simulink model "indy7_dualArm"  (R2024b)
settings: Solver=FixedStepAuto  StartTime=0.0  StopTime=10  FixedStep=0.001  RelTol=1e-3
model workspace (MAT data in the model file):
  joint_friction = [80 80 20 10 10 5]
  lambda_l_list = [0  -0.111945470246  -0.45  -0.23208429101  -0.00722667581655  -0.0911029490978  6.11257062428e-36; -1.17357539658  0.0246912114191  0  0.181466898367  -0.0447110760186  0.02862210596  -2.25514051877e-16; 0.993815552956  0.243747835972  -0.0305  0.141365128074  0.14506822671  0.174516399919  0.06; -2.091  1.20917417944  0  -1.20917417944  1.20917417944  -1.20917417944  0; 0  1.20917417944  0  -1.20905770917  1.20917417944  -1.20905770917  0; 0  -1.20905770917  0  1.20917417944  -1.20905770917  1.20917417944  0]
  lambda_r_list = [0  -0.111945470246  -0.45  -0.23208429101  -0.00722667581655  -0.0911029490978  -2.58853268681e-20; 1.17618914658  0.0246912114191  1.73472347598e-18  0.181466898367  -0.0447110760186  0.02862210596  2.25514051877e-16; 0.992300581915  0.243747835972  -0.0305  0.141365128074  0.14506822671  0.174516399919  0.06; 2.091  1.20917417944  1.04335921902e-16  -1.20917417944  1.20917417944  -1.20917417944  -1.83339582048e-16; 0  1.20917417944  -5.59082217244e-17  -1.20905770917  1.20917417944  -1.20905770917  -4.06575814682e-20; 0  -1.20905770917  1.31751732896e-17  1.20917417944  -1.20905770917  1.20917417944  0]
  lambda_rl_list = [2.58853268681e-20  0.0911029490978  0.00722667581655  0.23208429101  0.45  0.111945470246  0.701934663685  -0.111945470246  -0.45  -0.23208429101  -0.00722667581655  -0.0911029490978  2.43945488809e-21; -2.25514051877e-16  -0.02862210596  0.0447110760186  -0.181466898367  -1.73472347598e-18  -0.0246912114191  -0.00107834177066  0.0246912114191  -1.03338019565e-22  0.181466898367  -0.0447110760186  0.02862210596  -2.11636264069e-16; -0.06  -0.174516399919  -0.14506822671  -0.141365128074  0.0305  -0.243747835972  0.00061752626027  0.243747835972  -0.0305  0.141365128074  0.14506822671  0.174516399919  0.06; -1.83339582048e-16  1.20917417944  -1.20917417944  1.20917417944  1.04335921902e-16  -1.20917417944  -8.63118783402e-10  1.20917417944  0  -1.20917417944  1.20917417944  -1.20917417944  -2.89997910743e-16; -4.06575814682e-20  1.20905770917  -1.20917417944  1.20905770917  -5.59082217244e-17  -1.20917417944  2.72601580299  1.20917417944  -3.44383110592e-41  -1.20905770917  1.20917417944  -1.20905770917  -8.13151629364e-20; 0  -1.20917417944  1.20905770917  -1.20917417944  1.31751732896e-17  1.20905770917  -1.56154991477  -1.20905770917  0  1.20917417944  -1.20905770917  1.20917417944  0]
  q_init_l = Simulink.Parameter
  q_init_l.Value = [0.165747; 0.819274; 1.26369; 0.604148; 1.0515; -0.139217]
  q_init_l.Complexity = 'real'
  q_init_l.Dimensions = [6 1]
  q_init_l.DataType = 'double'
  q_init_l1 = Simulink.Parameter
  q_init_l1.Value = 0.165747
  q_init_l1.Complexity = 'real'
  q_init_l1.Dimensions = [1 1]
  q_init_l1.DataType = 'double'
  q_init_l2 = Simulink.Parameter
  q_init_l2.Value = 0.819274
  q_init_l2.Complexity = 'real'
  q_init_l2.Dimensions = [1 1]
  q_init_l2.DataType = 'double'
  q_init_l3 = Simulink.Parameter
  q_init_l3.Value = 1.26369
  q_init_l3.Complexity = 'real'
  q_init_l3.Dimensions = [1 1]
  q_init_l3.DataType = 'double'
  q_init_l4 = Simulink.Parameter
  q_init_l4.Value = 0.604148
  q_init_l4.Complexity = 'real'
  q_init_l4.Dimensions = [1 1]
  q_init_l4.DataType = 'double'
  q_init_l5 = Simulink.Parameter
  q_init_l5.Value = 1.0515
  q_init_l5.Complexity = 'real'
  q_init_l5.Dimensions = [1 1]
  q_init_l5.DataType = 'double'
  q_init_l6 = Simulink.Parameter
  q_init_l6.Value = -0.139217
  q_init_l6.Complexity = 'real'
  q_init_l6.Dimensions = [1 1]
  q_init_l6.DataType = 'double'
  q_init_r = Simulink.Parameter
  q_init_r.Value = [-0.165747; -0.819274; -1.26369; -0.604148; -1.0515; 0.139217]
  q_init_r.Complexity = 'real'
  q_init_r.Dimensions = [6 1]
  q_init_r.DataType = 'double'
  q_init_r1 = Simulink.Parameter
  q_init_r1.Value = -0.165747
  q_init_r1.Complexity = 'real'
  q_init_r1.Dimensions = [1 1]
  q_init_r1.DataType = 'double'
  q_init_r2 = Simulink.Parameter
  q_init_r2.Value = -0.819274
  q_init_r2.Complexity = 'real'
  q_init_r2.Dimensions = [1 1]
  q_init_r2.DataType = 'double'
  q_init_r3 = Simulink.Parameter
  q_init_r3.Value = -1.26369
  q_init_r3.Complexity = 'real'
  q_init_r3.Dimensions = [1 1]
  q_init_r3.DataType = 'double'
  q_init_r4 = Simulink.Parameter
  q_init_r4.Value = -0.604148
  q_init_r4.Complexity = 'real'
  q_init_r4.Dimensions = [1 1]
  q_init_r4.DataType = 'double'
  q_init_r5 = Simulink.Parameter
  q_init_r5.Value = -1.0515
  q_init_r5.Complexity = 'real'
  q_init_r5.Dimensions = [1 1]
  q_init_r5.DataType = 'double'
  q_init_r6 = Simulink.Parameter
  q_init_r6.Value = 0.139217
  q_init_r6.Complexity = 'real'
  q_init_r6.Dimensions = [1 1]
  q_init_r6.DataType = 'double'
  robot : robotics.RigidBodyTree (value not decoded)
values from neighbouring files (symbols this model uses):
  lambda_lr_list = [lambda_lr_list,-lambda_rl_list(:,i)]    [getDualArmLambdaList.m]    (also in untitled3.m)
  m = models{k}    [code_generation.m]
  N = length(q)    [FKLocalPOE.m]
undefined symbols (not defined in the file or in its folder): Blist_tcp, DiscIntNeverNeededParam, dt, exp6, M_tcp, q_init, q_max, q_min, qdot_max, qdot_min, SW_a, SW_b0, X, Y, Z
libraries: sm_lib x148, nesl_utility x45, robotmaniplib x9, robotcorelib x5, simulink x4, matrix_library x2
(part 1 of 5)
settings Model: Creator=sung  LastModifiedBy=sung
settings ExplorerConfigSet: InternalSimMechanicsExplorerSettings="<ExplorerConfiguration><canonicalview>default</canonicalview><AnimationSetting><BasePlaybackSpeed>1.0</BasePlaybackSpeed><PlaybackSpeedFactor>1.0</PlaybackSpeedFactor></AnimationSetting><TilePanel><TileInfo><Tiles Columns=\"1\" Count=\"1\" Rows=\"1\"><Column Weight=\"1\"/><Row Weight=\"1\"/><Tile Height=\"1\" Width=\"1\" X=\"0\" Y=\"0\"/></Tiles></TileInfo><SceneInfo><SceneViewer><BGColor><R>1</R><G>1</G><B>1</B></BGColor><Camera><DoPerspective>off</DoPerspective><Position><X>1.65343822930104345</X><Y>-0.838028370601997863</Y><Z>1.3090619282042868</Z></Position><Center><X>0.667257287193148252</X><Y>-0.49026343910033765</Y><Z>0.88933438419422528</Z></Center><Up><X>-0.446910653050087703</X><Y>-0.221156484844483803</Y><Z>0.866810635260998552</Z></Up><ViewLimDist>1</ViewLimDist><YLim>0.778338166596068581</YLim><XLim>1.03312002337695397</XLim></Camera></SceneViewer></SceneInfo></TilePanel><MechEditorPanel><Cameras/><GfxPanelCameraMap/><VideoCreator><PlaybackSpeedRatio>1.0</PlaybackSpeedRatio><FrameRate>30</FrameRate><VideoFormat>Motion JPEG AVI</VideoFormat><FrameSize>auto</FrameSize></VideoCreator></MechEditorPanel></ExplorerConfiguration>"

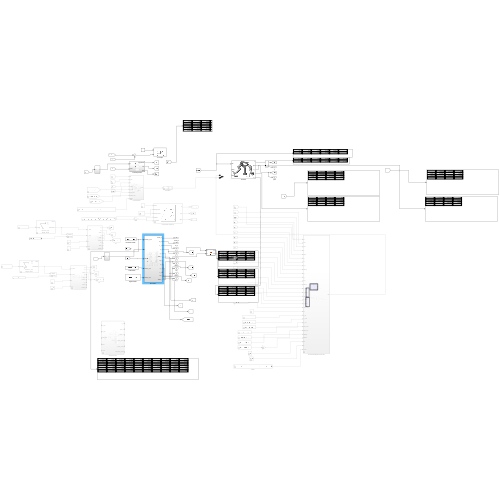
[thumbnail: Simulink's stored preview of the top-level diagram]
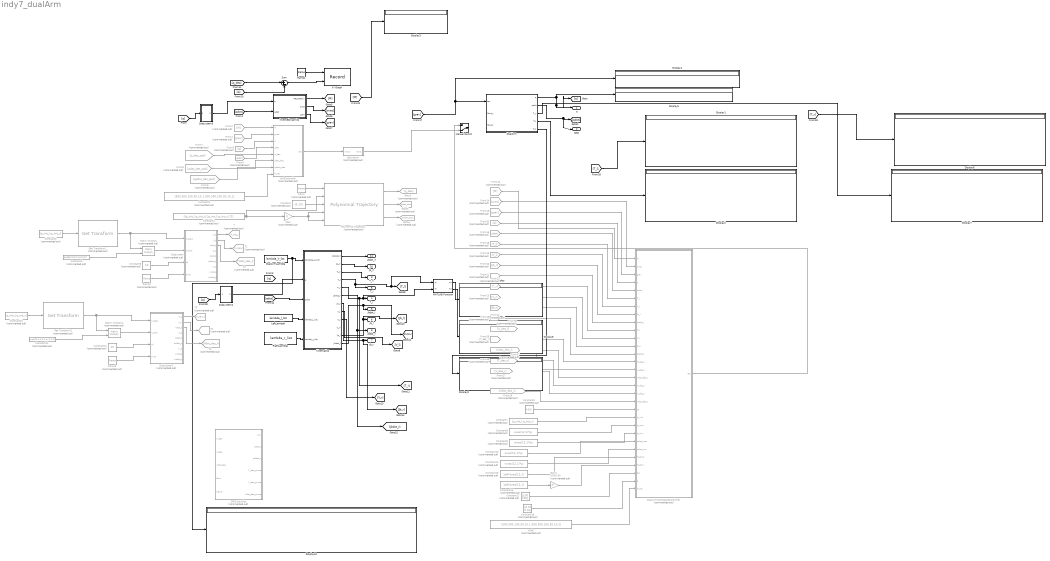
== system indy7_dualArm ==
  Constant : Constant  Commented=on  Value=[0,10]
  Constant1 : Constant  Commented=on  Value=[[q_init_l;q_init_r],[q_init_l;q_init_r].*2]
  Constant10 : Constant  Commented=on  Value=[q_init_l;q_init_r]
  Constant11 : Constant  Commented=on  Value=exp6([0.1,0,0.1,pi/2,0,0]')
  Constant12 : Constant  Commented=on  Value=10
  Constant13 : Constant  Commented=on  Value=ones(12,1)*pi
  Constant14 : Constant  Commented=on  Value=-ones(12,1)*pi
  Constant15 : Constant  Commented=on  Value=1e6*ones(12,1)
  Constant16 : Constant  Commented=on  Value=1e6*ones(12,1)
  Constant17 : Constant  Commented=on  Value=[100 100]
  Constant18 : Constant  Commented=on  Value=[0.01 0.01]
  Constant2 : Constant  Commented=on  Value=[500,500,100,50,10,1,500,500,100,50,10,1]
  Constant3 : Constant  Commented=on  Value=[q_init_l;q_init_r]
  Constant4 : Constant  Commented=on  Value=exp6([0,0,0.1,0,0,0]')
  Constant5 : Constant  Commented=on  Value=10
  Constant6 : Constant  Commented=on  Value=0.001
  Constant7 : Constant  Commented=on  Value=[q_init_l;q_init_r]
  Constant8 : Constant  Commented=on  Value=ones(12,1)*pi
  Constant9 : Constant  Commented=on  Value=-ones(12,1)*pi
  Display{,1..10} (11 alike) : Display
  DualArm : Subsystem
      mask Display: image('dualarm.png');
  DualArmLambda : Constant  Value=lambda_lr_list
  DualArmTaskSpaceController : Subsystem  Commented=on
  From13 : From  Commented=on  GotoTag=M
  From14 : From  Commented=on  GotoTag=cvec
  From15 : From  Commented=on  GotoTag=grav
  From16 : From  Commented=on  GotoTag=qdot
  From18 : From  Commented=on  GotoTag=T_l
  From19 : From  Commented=on  GotoTag=V_l
  From2 : From  Commented=on  GotoTag=M
  From20 : From  Commented=on  GotoTag=Jb_l
  From21 : From  Commented=on  GotoTag=Jbdot_l
  From22 : From  Commented=on  GotoTag=T_r
  From23 : From  Commented=on  GotoTag=V_r
  From24 : From  Commented=on  GotoTag=Jb_r
  From25 : From  Commented=on  GotoTag=Jbdot_r
  From26 : From  Commented=on  GotoTag=T_des_l
  From27 : From  Commented=on  GotoTag=V_des_r
  From29 : From  Commented=on  GotoTag=Vdot_des_r
  From32 : From  Commented=on  GotoTag=q
  From36 : From  Commented=on  GotoTag=V_des_l
  From37 : From  Commented=on  GotoTag=Vdot_des_l
  From38 : From  Commented=on  GotoTag=T_des_r
  From4 : From  Commented=on  GotoTag=grav
  From5 : From  Commented=on  GotoTag=q
  From6 : From  Commented=on  GotoTag=qdot
  From7 : From  Commented=on  GotoTag=q_des_spd
  From8 : From  Commented=on  GotoTag=qdot_des_spd
  From9 : From  Commented=on  GotoTag=qddot_des_spd
  Gain : Gain  Commented=on  Gain=0
  Gain1 : Gain  Commented=on  Gain=0.001*30
  Get Transform1 : robotmaniplib/Get Transform  Commented=on  RigidBodyTree=robot  SourceBody=l_tcp  TargetBody=world  SimulateUsing=Code generation
  Get Transform2 : robotmaniplib/Get Transform  Commented=on  RigidBodyTree=robot  SourceBody=r_tcp  TargetBody=world  SimulateUsing=Code generation
  Goto2 : Goto  Commented=on  GotoTag=q_des
  Goto3 : Goto  Commented=on  GotoTag=qdot_des
  Goto4 : Goto  Commented=on  GotoTag=qddot_des
  HInfController : Subsystem  Commented=on
  HinfK : Constant  Commented=on  Value=[500,500,100,50,10,1,500,500,100,50,10,1]
  InverseDynamics : Subsystem
  Kinematics : Subsystem
  LeftLambda : Constant  Value=lambda_l_list
  MATLAB Function : MATLAB Function  TreatAsAtomicUnit=on
  Manual Switch : ManualSwitch  CurrentSetting=0
  Matrix Multiply : Product  Commented=on  Multiplication=Matrix(*)
  Matrix Multiply1 : Product  Commented=on  Multiplication=Matrix(*)
  Polynomial Trajectory : robotcorelib/Polynomial Trajectory  Commented=on  WaypointSource=External  Waypoints=[ 0, 2, 1, 5, 0; -1, 3, 1, 4, 4 ]  TimePoints=[ 0, 1, 2, 3, 4 ]  TimeInterval=[ 1, 4 ]  Method=Quintic Polynomial  ParameterSource=External  VelocityBoundaryCondition=zeros( 2, 5 )  AccelerationBoundaryCondition=zeros( 2, 5 )  SimulateUsing=Interpreted execution
  Ramp : simulink/Sources/Ramp  Commented=on  slope=1  start=0  InitialOutput=0
  Ramp1 : simulink/Sources/Ramp  slope=1  start=0  InitialOutput=0
  Ramp2 : simulink/Sources/Ramp  Commented=on  slope=1  start=0  InitialOutput=0
  Ramp3 : simulink/Sources/Ramp  Commented=on  slope=1  start=0  InitialOutput=0
  RightLambda : Constant  Value=lambda_r_list
  SPDController : Subsystem  Commented=on
  Saturation : Subsystem  Commented=on
  Subsystem : Subsystem  Commented=on
  Subsystem1 : Subsystem  Commented=on
  Subsystem2 : Subsystem
  Subsystem3 : Subsystem
  Sum : Sum  Inputs=|+-
  T : Goto  Commented=on  GotoTag=T_des_l
  T1 : Goto  Commented=on  GotoTag=V_des_l
  T2 : Goto  Commented=on  GotoTag=Vdot_des_l
  T3 : Goto  Commented=on  GotoTag=T_des_r
  T4 : Goto  Commented=on  GotoTag=V_des_r
  T5 : Goto  Commented=on  GotoTag=Vdot_des_r
  XY Graph : Record  FileSettingsInternal="{\"entries\":[{\"content\":{\"excelSettings\":{\"content\":{},\"type\":\"Streamout.ExcelSettings\"}},\"type\":\"Streamout.FileSettingStorage\",\"uuid\":\"\"}],\"packageUris\":[\"http:\\/\\/schema.mathworks.com\\/mf0\\/streamout_blocks\\/R2020a\"],\"version\":\"1.0\"}"  Layout=[1 1]  SignalsInternal="{\"entries\":[{\"content\":{\"signals\":[{\"content\":{\"blockPath\":[],\"dimensions\":[1],\"domain\":\"\",\"lineColor\":\"#a2142f\",\"plots\":[ 1 ],\"port\":1,\"sid\":[\"\"],\"signalID\":1,\"signalName\":\"Ramp1\"},\"type\":\"RecordBlkView.Signal\",\"uuid\":\"\"},{\"content\":{\"blockPath\":[],\"dimensions\":[12],\"domain\":\"\",\"hasChildren\":true,\"lineColor\":\"#77ac30\",\"lineWidth\":2,\"port\":2,\"sid\":[\"\"],\"signalID\":2,\"signalName\":\"Sum\"},\"type\":\"RecordBlkView.Signal\",\"uuid\":\"\"},{\"content\":{\"blockPath\":[],\"channel\":[1],\"dimensions\":[12],\"domain\":\"\",\"lineColor\":\"#77ac30\",\"lineWidth\":2,\"parentID\":2,\"port\":2,\"sid\":[\"\"],\"signalID\":3,\"signalName\":\"Sum\"},\"type\":\"RecordBlkView.Signal\",\"uuid\":\"\"}]},\"type\":\"RecordBlkView.InputSignals\",\"uuid\":\"\"}],\"packageUris\":[\"http:\\/\\/schema.mathworks.com\\/mf0\\/streamout_blocks\\/R2020a\"],\"version\":\"1.0\"}"  VisualizationBindings="{\"xyplotplugin\":{\"info\":[{\"series\":[{\"bindingParametersList\":[{\"parameter\":\"X-Axis\",\"signalID\":1,\"signalName\":\"Ramp1\"}],\"seriesID\":0},{\"bindingParametersList\":[{\"parameter\":\"X-Axis\",\"signalID\":1,\"signalName\":\"Ramp1\"}],\"seriesID\":1},{\"bindingParametersList\":[{\"parameter\":\"X-Axis\",\"signalID\":1,\"signalName\":\"Ramp1\"}],\"seriesID\":2},{\"bindingParametersList\":[{\"parameter\":\"X-Axis\",\"signalID\":1,\"signalName\":\"Ramp1\"}],\"seriesID\":3},{\"bindingParametersList\":[{\"parameter\":\"X-Axis\",\"signalID\":1,\"signalName\":\"Ramp1\"}],\"seriesID\":4},{\"bindingParametersList\":[{\"parameter\":\"X-Axis\",\"signalID\":1,\"signalName\":\"Ramp1\"}],\"seriesID\":5},{\"bindingParametersList\":[{\"parameter\":\"X-Axis\",\"signalID\":1,\"signalName\":\"Ramp1\"}],\"seriesID\":6},{\"bindingParametersList\":[{\"parameter\":\"X-Axis\",\"signalID\":1,\"signalName\":\"Ramp1\"}],\"seriesID\":7},{\"bindingParametersList\":[{\"parameter\":\"X-Axis\",\"signalID\":1,\"signalName\":\"Ramp1\"}],\"seriesID\":8},{\"bindingParametersList\":[{\"parameter\":\"X-Axis\",\"signalID\":1,\"signalName\":\"Ramp1\"}],\"seriesID\":9},{\"bindingParametersList\":[{\"parameter\":\"X-Axis\",\"signalID\":1,\"signalName\":\"Ramp1\"}],\"seriesID\":10}],\"subplotID\":1}]}}"  CompatibilityTag=XY
  q : Outport
  qdot : Outport  Port=2
  T_rl : Outport  Port=3
  T_r : Outport  Port=4
  T_l : Outport  Port=5
  Jb_l : Outport  Port=6
  Jb_r : Outport  Port=7
  Jbdot_l : Outport  Port=8
  Jbdot_r : Outport  Port=9
  Jb_rl : Outport  Port=10
  Jbdot_rl : Outport  Port=11
  wires:
  InverseDynamics/3(grav) -> [grav]
  [q_des] -> Sum/1
  From2/1 -> HInfController/1(M)
  DualArm/2(qdot) -> qdot/1, [qdot]
  [q] -> Sum/2
  From5/1 -> HInfController/3(q)
  [qdot] -> InverseDynamics/2(qdot)
  From4/1 -> HInfController/2(gvec)
  From6/1 -> HInfController/4(qdot)
  From7/1 -> HInfController/5(q_des)
  From8/1 -> HInfController/6(qdot_des)
  From9/1 -> HInfController/7(qddot_des)
  InverseDynamics/1(MassMatrix) -> [M]
  Constant1/1 -> Polynomial Trajectory/2, Gain/1
  Constant2/1 -> HInfController/8(HinfK)
  Ramp1/1 -> XY Graph/1
  Sum/1 -> XY Graph/2
  InverseDynamics/2(cvec) -> [cvec]
  HInfController/1(tau) -> Saturation/1(Input)
  Ramp/1 -> Polynomial Trajectory/1
  Polynomial Trajectory/2 -> Goto3/1
  Constant/1 -> Polynomial Trajectory/3
  Gain/1 -> Polynomial Trajectory/5, Polynomial Trajectory/4
  Polynomial Trajectory/1 -> Goto2/1
  Polynomial Trajectory/3 -> Goto4/1
  DualArm/1(q) -> [q], q/1, Display5/1
  DualArmLambda/1 -> Display10/1, Kinematics/1(lambda_lr_list)
  [qdot] -> Kinematics/3(qdot)
  Kinematics/1(Jbdot_lrl) -> Jbdot_rl/1
  Kinematics/2(Jb_lr) -> Jb_rl/1
  Kinematics/3(T_lr) -> T_rl/1
  Kinematics/4(T_l) -> T_l/1, MATLAB Function/1(Tl), [T_l]
  Kinematics/5(T_r) -> [T_r], MATLAB Function/2(Tr), T_r/1
  Kinematics/12(Jbdot_l) -> Jbdot_l/1, [Jbdot_l]
  Kinematics/11(Jb_l) -> [Jb_l], Jb_l/1
  Kinematics/6(Jbdot_r) -> [Jbdot_r], Jbdot_r/1
  Kinematics/7(Jb_r) -> [Jb_r], Jb_r/1
  LeftLambda/1 -> Kinematics/4(lamba_l_list)
  RightLambda/1 -> Kinematics/5(lamba_r_list)
  Constant3/1 -> Get Transform1/1
  Get Transform1/1 -> Matrix Multiply/1, Subsystem/1(T_start)
  Constant4/1 -> Matrix Multiply/2
  Matrix Multiply/1 -> Subsystem/2(T_end)
  Constant5/1 -> Subsystem/3(Tf)
  Ramp2/1 -> Subsystem/4(time)
  Subsystem/1(T_t) -> T/1
  Subsystem/2(V_t) -> T1/1
  Subsystem/3(Vdot_t) -> T2/1
  Kinematics/8(V_l) -> [V_l]
  Subsystem1/2(V_t) -> T4/1
  Ramp3/1 -> Subsystem1/4(time)
  Subsystem1/3(Vdot_t) -> T5/1
  Constant10/1 -> Get Transform2/1
  Matrix Multiply1/1 -> Subsystem1/2(T_end)
  Constant11/1 -> Matrix Multiply1/2
  Get Transform2/1 -> Matrix Multiply1/1, Subsystem1/1(T_start)
  Constant12/1 -> Subsystem1/3(Tf)
  Subsystem1/1(T_t) -> T3/1
  Kinematics/9(V_r) -> [V_r]
  Saturation/1(Out1) -> Manual Switch/2
  From13/1 -> DualArmTaskSpaceController/1(M)
  From14/1 -> DualArmTaskSpaceController/2(cvec)
  From15/1 -> DualArmTaskSpaceController/3(grav)
  From32/1 -> DualArmTaskSpaceController/4(q)
  From16/1 -> DualArmTaskSpaceController/5(qdot)
  Constant6/1 -> DualArmTaskSpaceController/20(dt)
  From18/1 -> DualArmTaskSpaceController/6(T_l)
  From19/1 -> DualArmTaskSpaceController/7(V_l)
  From20/1 -> DualArmTaskSpaceController/8(Jb_l)
  From21/1 -> DualArmTaskSpaceController/9(Jbdot_l)
  From22/1 -> DualArmTaskSpaceController/10(T_r)
  From23/1 -> DualArmTaskSpaceController/11(V_r)
  From24/1 -> DualArmTaskSpaceController/12(Jb_r)
  From25/1 -> DualArmTaskSpaceController/13(Jbdot_r)
  From26/1 -> DualArmTaskSpaceController/14(T_des_l)
  From36/1 -> DualArmTaskSpaceController/15(V_des_l)
  From37/1 -> DualArmTaskSpaceController/16(Vdot_des_l)
  From38/1 -> DualArmTaskSpaceController/17(T_des_r)
  From27/1 -> DualArmTaskSpaceController/18(V_des_r)
  From29/1 -> DualArmTaskSpaceController/19(Vdot_des_r)
  Constant7/1 -> DualArmTaskSpaceController/21(q_init)
  Constant8/1 -> DualArmTaskSpaceController/22(q_max)
  Constant9/1 -> DualArmTaskSpaceController/23(q_min)
  Constant13/1 -> DualArmTaskSpaceController/24(qdot_max)
  Constant14/1 -> DualArmTaskSpaceController/25(qdot_min)
  Constant15/1 -> DualArmTaskSpaceController/26(TaskKp)
  Constant16/1 -> Gain1/1
  Gain1/1 -> DualArmTaskSpaceController/27(TaskKv)
  Constant17/1 -> DualArmTaskSpaceController/28(b0)
  Constant18/1 -> DualArmTaskSpaceController/29(a)
  HinfK/1 -> DualArmTaskSpaceController/30(HinfK)
  DualArmTaskSpaceController/1(tau) -> Manual Switch/1
  MATLAB Function/1(Tlr) -> Display/1
  [grav] -> Display4/1, DualArm/1(tau)
  [T_l] -> Display1/1
  DualArm/4(T_l) -> Display2/1
  [q] -> Subsystem2/1(In1)
  Subsystem2/1(Out1) -> Kinematics/2(q)
  [M] -> Display3/1
  [q] -> Subsystem3/1(In1)
  Subsystem3/1(Out1) -> InverseDynamics/1(q)
  [T_r] -> Display6/1
  DualArm/3(T_r) -> Display7/1
  MATLAB Function/2(Trl) -> Display8/1
  DualArm/5(T_rl) -> Display9/1

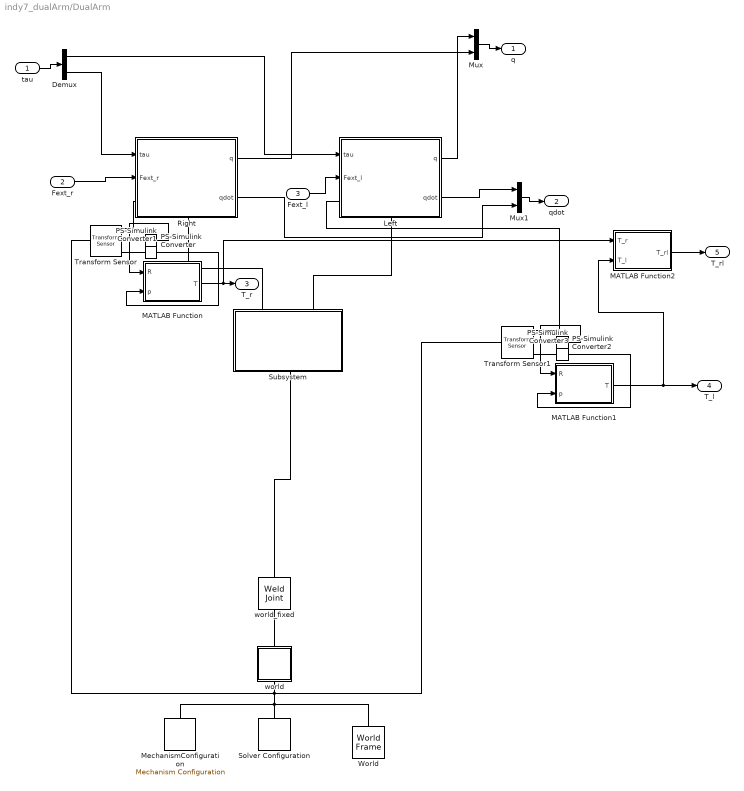
== system indy7_dualArm/DualArm ==
  tau : Inport
  Fext_r : Inport  Port=2
  Fext_l : Inport  Port=3
  Demux : Demux  Outputs=2
  Left : Subsystem
      settings: PortSchema="{\"entries\":[{\"content\":{\"sides\":[{\"content\":{\"connectorIds\":[\"In1\",\"In2\",\"LConn1\"]},\"type\":\"ConnectorPlacement.EquallySpacedRectSide\",\"uuid\":\"a802bf1d-865c-44a2-b0f5-a6da758969a6\"},{\"content\":{\"connectorIds\":[\"Out1\",\"Out2\"],\"side\":\"RIGHT\"},\"type\":\"ConnectorPlacement.EquallySpacedRectSide\",\"uuid\":\"5f6dd1c3-913e-4ce9-9167-95590779c30f\"},{\"content\":{\"side\":\"TOP\"},\"type\":\"ConnectorPlacement.EquallySpacedRectSide\",\"uuid\":\"64c6b8e9-73c0-45a3-a4f2-c2cb7725a77f\"},{\"content\":{\"connectorIds\":[\"RConn1\"],\"side\":\"BOTTOM\"},\"type\":\"ConnectorPlacement.EquallySpacedRectSide\",\"uuid\":\"95edfb6b-d02c-40cc-a449-2c9849400bda\"}]},\"type\":\"ConnectorPlacement.EquallySpacedConnector\",\"uuid\":\"45caad31-32a3-4e19-8c7b-99b9e1313351\"}],\"packageUris\":[\"http://schema.mathworks.com/mf0/Connector/R2020b\"],\"version\":\"1.0\"}"
  MATLAB Function : MATLAB Function  TreatAsAtomicUnit=on
  MATLAB Function1 : MATLAB Function  TreatAsAtomicUnit=on
  MATLAB Function2 : MATLAB Function  TreatAsAtomicUnit=on
  MechanismConfiguration : sm_lib/Utilities/Mechanism Configuration  UniformGravity=Constant  GravityVector=[0 0 -9.80665]  GravityVectorUnits=m/s^2  LinearizationDelta=0.001  JointModeTransitionNonlinearIterations=2
  Mux : Mux  Inputs=2
  Mux1 : Mux  Inputs=2
  PS-Simulink Converter{,1..3} (4 alike) : nesl_utility/PS-Simulink Converter  PhysicalDomain=network_engine_domain  SubClassName=ps_output  LeftPortType=input  RightPortType=output  PseudoPeriodic=off  Frequencies=[]  VectorFormat=inherit  Unit=inherit  AffineConversion=off
  Right : Subsystem
      settings: PortSchema="{\"entries\":[{\"content\":{\"sides\":[{\"content\":{\"connectorIds\":[\"In1\",\"In2\",\"LConn1\"]},\"type\":\"ConnectorPlacement.EquallySpacedRectSide\",\"uuid\":\"fdf178f2-e7c3-4173-86ca-7321804fb5d5\"},{\"content\":{\"connectorIds\":[\"Out1\",\"Out2\"],\"side\":\"RIGHT\"},\"type\":\"ConnectorPlacement.EquallySpacedRectSide\",\"uuid\":\"59022458-aa9c-4c83-9b4f-7726f2382bb8\"},{\"content\":{\"side\":\"TOP\"},\"type\":\"ConnectorPlacement.EquallySpacedRectSide\",\"uuid\":\"4f63f239-705d-4500-8a4d-d984146f717c\"},{\"content\":{\"connectorIds\":[\"RConn1\"],\"side\":\"BOTTOM\"},\"type\":\"ConnectorPlacement.EquallySpacedRectSide\",\"uuid\":\"092b85dc-93e6-45d5-b73f-7a2a4320a625\"}]},\"type\":\"ConnectorPlacement.EquallySpacedConnector\",\"uuid\":\"427c422a-fe45-4c4a-9206-8f07c894b426\"}],\"packageUris\":[\"http://schema.mathworks.com/mf0/Connector/R2020b\"],\"version\":\"1.0\"}"
  Solver Configuration : nesl_utility/Solver Configuration  PhysicalDomain=network_engine_domain  SubClassName=solver  LeftPortType=input  RightPortType=generic  Tones=[]  Harmonics=[]  SimulateNoise=off  Profile=off  UseLocalSampling=off  EnableSwitchedLinearOptims=on  FrequencyDomain=off  UseCCode=off  RelTol=0.001  AbsTol=0.001  MinStep=1e-09  ToWorkspace=off  RevertToSquareIcSolve=off  NumHomotopyIterations=100  PhasorMode=off  PhasorModeNumHarmonics=1  ConsistencySolver=NEWTON_XTOL_AFTER_FTOL  IndexReductionMethod=DerivativeReplacement  DoDC=off  ResidualTolerance=1e-09  ConsistencyTolSource=GLOBAL  ConsistencyAbsTol=0.001  ConsistencyRelTol=0.001  ConsistencyTolFactor=0.001  UseLocalSolver=off  LocalSolverChoice=NE_BACKWARD_EULER_ADVANCER  ResolveIndetEquations=on  FunctionEvalNumThread=1  LocalSolverSampleTime=0.001  DoFixedCost=off  MaxNonlinIter=3  MaxModeIter=2  ComputeImpulses=off  ImpulseIterations=2  LinearAlgebra=auto  LinearAlgebraNumThread=0  EquationFormulation=NE_TIME_EF  DelaysMemoryBudget=1024  AutomaticFiltering=on  FilteringTimeConstant=0.001  PartitionStorageMethod=AS_NEEDED  PartitionMemoryBudget=1024  PartitionMethod=ROBUST  MultibodyUseLocalSolver=on  MultibodyLocalSolverChoice=ODE1  MultibodyLocalSolverSampleTime=0.001
  Subsystem : Subsystem
  Transform Sensor : sm_lib/Frames and Transforms/Transform Sensor  MeasurementFrame=World  RotationSequence=XYX  SenseAngle=off  SenseAxis=off  SenseQ=off  SenseR=on  SenseRotationSequence=off  SenseOmegaX=off  SenseOmegaY=off  SenseOmegaZ=off  SenseOmega=off  SenseQDot=off  SenseRDot=off  SenseRotationSequenceDot=off  SenseAlphaX=off  SenseAlphaY=off  SenseAlphaZ=off  SenseAlpha=off  SenseQDDot=off  SenseRDDot=off  SenseX=off  SenseY=off  SenseZ=off  SenseXYZ=on  SenseRad=off  SenseAzim=off  SenseDist=off  SenseInc=off  SenseXDot=off  SenseYDot=off  SenseZDot=off  SenseXYZDot=off  SenseRadDot=off  SenseAzimDot=off  SenseDistDot=off  SenseIncDot=off  SenseXDDot=off  SenseYDDot=off  SenseZDDot=off  SenseXYZDDot=off  SenseRadDDot=off  SenseAzimDDot=off  SenseDistDDot=off  SenseIncDDot=off
  Transform Sensor1 : sm_lib/Frames and Transforms/Transform Sensor  MeasurementFrame=World  RotationSequence=XYX  SenseAngle=off  SenseAxis=off  SenseQ=off  SenseR=on  SenseRotationSequence=off  SenseOmegaX=off  SenseOmegaY=off  SenseOmegaZ=off  SenseOmega=off  SenseQDot=off  SenseRDot=off  SenseRotationSequenceDot=off  SenseAlphaX=off  SenseAlphaY=off  SenseAlphaZ=off  SenseAlpha=off  SenseQDDot=off  SenseRDDot=off  SenseX=off  SenseY=off  SenseZ=off  SenseXYZ=on  SenseRad=off  SenseAzim=off  SenseDist=off  SenseInc=off  SenseXDot=off  SenseYDot=off  SenseZDot=off  SenseXYZDot=off  SenseRadDot=off  SenseAzimDot=off  SenseDistDot=off  SenseIncDot=off  SenseXDDot=off  SenseYDDot=off  SenseZDDot=off  SenseXYZDDot=off  SenseRadDDot=off  SenseAzimDDot=off  SenseDistDDot=off  SenseIncDDot=off
  World : sm_lib/Frames and Transforms/World Frame
  world : Subsystem
  world_fixed : sm_lib/Joints/Weld Joint  JointMode=Normal  CompositeWrenchDir=FollowerOnBase  CompositeWrenchFrame=BaseFrame  SenseConstraintForce=off  SenseConstraintTorque=off  SenseTotalForce=off  SenseTotalTorque=off
  q : Outport
  qdot : Outport  Port=2
  T_r : Outport  Port=3
  T_l : Outport  Port=4
  T_rl : Outport  Port=5
  wires:
  tau/1 -> Demux/1
  Left/1(q) -> Mux/1
  Mux/1 -> q/1
  Demux/2 -> Right/1(tau)
  Left/2(qdot) -> Mux1/1
  Mux1/1 -> qdot/1
  Right/1(q) -> Mux/2
  Right/2(qdot) -> Mux1/2
  Demux/1 -> Left/1(tau)
  PS-Simulink Converter/1 -> MATLAB Function/1(R)
  PS-Simulink Converter1/1 -> MATLAB Function/2(p)
  MATLAB Function/1(T) -> MATLAB Function2/1(T_r), T_r/1
  PS-Simulink Converter2/1 -> MATLAB Function1/1(R)
  PS-Simulink Converter3/1 -> MATLAB Function1/2(p)
  MATLAB Function1/1(T) -> MATLAB Function2/2(T_l), T_l/1
  MATLAB Function2/1(T_rl) -> T_rl/1
  Fext_r/1 -> Right/2(Fext_r)
  Fext_l/1 -> Left/2(Fext_l)
  connections:
  world/RConn1 -- world_fixed/LConn1
  Transform Sensor/LConn1 -- world/LConn1 -- Solver Configuration/RConn1 -- World/RConn1 -- MechanismConfiguration/RConn1 -- Transform Sensor1/LConn1
  world_fixed/RConn1 -- Subsystem/LConn1
  Subsystem/RConn1 -- Right/RConn1
  PS-Simulink Converter/LConn1 -- Transform Sensor/RConn2
  PS-Simulink Converter1/LConn1 -- Transform Sensor/RConn3
  Transform Sensor/RConn1 -- Right/LConn1
  PS-Simulink Converter3/LConn1 -- Transform Sensor1/RConn3
  PS-Simulink Converter2/LConn1 -- Transform Sensor1/RConn2
  Transform Sensor1/RConn1 -- Left/LConn1
  Subsystem/RConn2 -- Left/RConn1

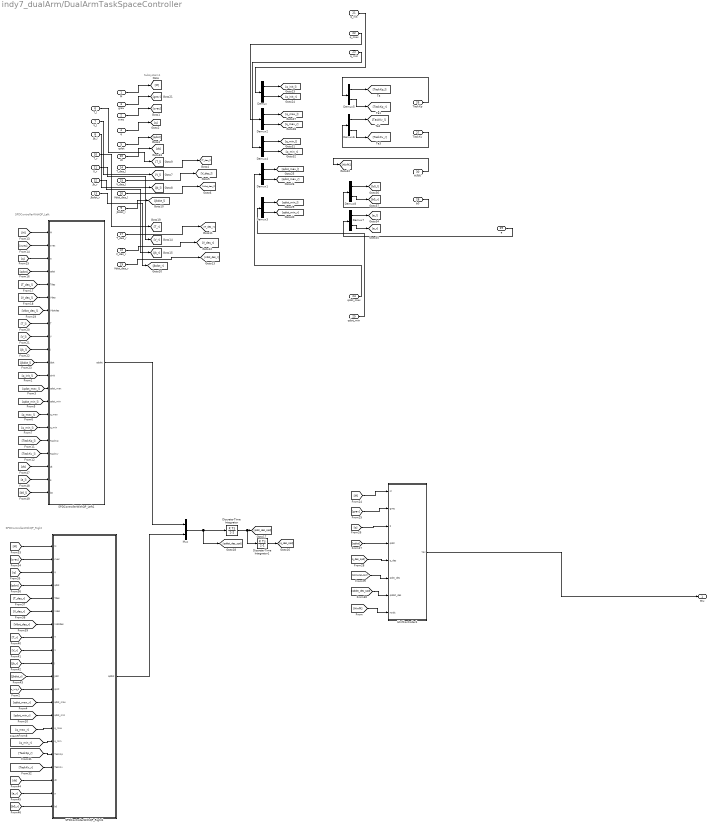
== system indy7_dualArm/DualArmTaskSpaceController ==
  note: SPDControllerWithQP_Right
  note: SPDControllerWithQP_Left
  note: Subsystem1
  M : Inport
  cvec : Inport  Port=2
  grav : Inport  Port=3
  q : Inport  Port=4
  qdot : Inport  Port=5
  T_l : Inport  Port=6
  V_l : Inport  Port=7
  Jb_l : Inport  Port=8
  Jbdot_l : Inport  Port=9
  T_r : Inport  Port=10
  V_r : Inport  Port=11
  Jb_r : Inport  Port=12
  Jbdot_r : Inport  Port=13
  T_des_l : Inport  Port=14
  V_des_l : Inport  Port=15
  Vdot_des_l : Inport  Port=16
  T_des_r : Inport  Port=17
  V_des_r : Inport  Port=18
  Vdot_des_r : Inport  Port=19
  dt : Inport  Port=20
  q_init : Inport  Port=21
  q_max : Inport  Port=22
  q_min : Inport  Port=23
  qdot_max : Inport  Port=24
  qdot_min : Inport  Port=25
  TaskKp : Inport  Port=26
  TaskKv : Inport  Port=27
  b0 : Inport  Port=28
  a : Inport  Port=29
  HinfK : Inport  Port=30
  Demux{,1..8} (9 alike) : Demux  Outputs=2
  Discrete-Time Integrator : DiscreteIntegrator  SampleTime=-1  UpperSaturationLimit=ones(12,1)*pi  LowerSaturationLimit=-ones(12,1)*pi  ICPrevOutput=DiscIntNeverNeededParam  ICPrevScaledInput=DiscIntNeverNeededParam
  Discrete-Time Integrator1 : DiscreteIntegrator  InitialCondition=[q_init_l;q_init_r]  SampleTime=-1  UpperSaturationLimit=ones(12,1)*3.054325556  LowerSaturationLimit=-ones(12,1)*3.054325556  ICPrevOutput=DiscIntNeverNeededParam  ICPrevScaledInput=DiscIntNeverNeededParam
  HInfController1 : Subsystem
  Mux : Mux  Inputs=2
  SPDControllerWithQP_Left1 : MATLAB Function  TreatAsAtomicUnit=on
  SPDControllerWithQP_Right1 : MATLAB Function  TreatAsAtomicUnit=on
  tau : Outport
  wires:
  HInfController1/1(tau) -> tau/1
  Demux/1 -> [q_init_l]
  Demux1/2 -> [qdot_max_r]
  Demux1/1 -> [qdot_max_l]
  Demux7/2 -> [a_r]
  Demux2/1 -> [q_max_l]
  Demux7/1 -> [a_l]
  qdot_max/1 -> Demux1/1
  Demux2/2 -> [q_max_r]
  V_des_r/1 -> [V_des_r]
  T_des_r/1 -> [T_des_r]
  TaskKp/1 -> Demux5/1
  qdot/1 -> [qdot]
  HinfK/1 -> [HinfK]
  T_des_l/1 -> [T_des_l]
  T_l/1 -> [T_l]
  Demux4/1 -> [q_min_l]
  Demux4/2 -> [q_min_r]
  Jbdot_r/1 -> [Jbdot_r]
  T_r/1 -> [T_r]
  Demux8/1 -> [b0_l]
  Demux8/2 -> [b0_r]
  Vdot_des_r/1 -> [Vdot_des_r]
  V_r/1 -> [V_r]
  Demux/2 -> [q_init_r]
  qdot_min/1 -> Demux3/1
  V_des_l/1 -> [V_des_l]
  Demux5/2 -> [TaskKp_r]
  Demux6/2 -> [TaskKv_r]
  Demux6/1 -> [TaskKv_l]
  q/1 -> [q]
  M/1 -> [M]
  Demux3/2 -> [qdot_min_r]
  Demux3/1 -> [qdot_min_l]
  Demux5/1 -> [TaskKp_l]
  TaskKv/1 -> Demux6/1
  Vdot_des_l/1 -> [Vdot_des_l]
  Jb_r/1 -> [Jb_r]
  dt/1 -> [dt]
  Jbdot_l/1 -> [Jbdot_l]
  grav/1 -> [grav]
  q_init/1 -> Demux/1
  q_max/1 -> Demux2/1
  V_l/1 -> [V_l]
  q_min/1 -> Demux4/1
  b0/1 -> Demux8/1
  Jb_l/1 -> [Jb_l]
  cvec/1 -> [cvec]
  a/1 -> Demux7/1
  [q] -> HInfController1/3(q)
  [qddot_des_spd] -> HInfController1/7(qddot_des)
  [q_des_spd] -> HInfController1/5(q_des)
  [qdot] -> HInfController1/4(qdot)
  [M] -> HInfController1/1(M)
  [qdot_des_spd] -> HInfController1/6(qdot_des)
  [HinfK] -> HInfController1/8(HinfK)
  Mux/1 -> Discrete-Time Integrator/1, [qddot_des_spd]
  SPDControllerWithQP_Left1/1(qddot) -> Mux/1
  Discrete-Time Integrator/1 -> Discrete-Time Integrator1/1, [qdot_des_spd]
  Discrete-Time Integrator1/1 -> [q_des_spd]
  [grav] -> HInfController1/2(gvec)
  SPDControllerWithQP_Right1/1(qddot) -> Mux/2
  [M] -> SPDControllerWithQP_Left1/1(M)
  [cvec] -> SPDControllerWithQP_Left1/2(cvec)
  [T_des_l] -> SPDControllerWithQP_Left1/5(Tdes)
  [qdot] -> SPDControllerWithQP_Left1/4(qdot)
  [V_des_l] -> SPDControllerWithQP_Left1/6(Vdes)
  [Vdot_des_l] -> SPDControllerWithQP_Left1/7(Vdotdes)
  [q_min_l] -> SPDControllerWithQP_Left1/16(q_min)
  [T_l] -> SPDControllerWithQP_Left1/8(T)
  [q_init_l] -> SPDControllerWithQP_Left1/12(qinit)
  [V_l] -> SPDControllerWithQP_Left1/9(V)
  [q] -> SPDControllerWithQP_Left1/3(q)
  [Jb_l] -> SPDControllerWithQP_Left1/10(J)
  [TaskKp_l] -> SPDControllerWithQP_Left1/17(TaskKp)
  [qdot_min_l] -> SPDControllerWithQP_Left1/14(qdot_min)
  [dt] -> SPDControllerWithQP_Left1/19(dt)
  [qdot_max_l] -> SPDControllerWithQP_Left1/13(qdot_max)
  [q_max_l] -> SPDControllerWithQP_Left1/15(q_max)
  [a_l] -> SPDControllerWithQP_Left1/20(a)
  [TaskKv_l] -> SPDControllerWithQP_Left1/18(TaskKv)
  [Jbdot_l] -> SPDControllerWithQP_Left1/11(Jdot)
  [b0_l] -> SPDControllerWithQP_Left1/21(b0)
  [M] -> SPDControllerWithQP_Right1/1(M)
  [q] -> SPDControllerWithQP_Right1/3(q)
  [qdot] -> SPDControllerWithQP_Right1/4(qdot)
  [cvec] -> SPDControllerWithQP_Right1/2(cvec)
  [b0_r] -> SPDControllerWithQP_Right1/21(b0)
  [qdot_min_r] -> SPDControllerWithQP_Right1/14(qdot_min)
  [V_r] -> SPDControllerWithQP_Right1/9(V)
  [Vdot_des_r] -> SPDControllerWithQP_Right1/7(Vdotdes)
  [q_max_r] -> SPDControllerWithQP_Right1/15(q_max)
  [q_min_r] -> SPDControllerWithQP_Right1/16(q_min)
  [T_r] -> SPDControllerWithQP_Right1/8(T)
  [T_des_r] -> SPDControllerWithQP_Right1/5(Tdes)
  [q_init_r] -> SPDControllerWithQP_Right1/12(qinit)
  [Jbdot_r] -> SPDControllerWithQP_Right1/11(Jdot)
  [Jb_r] -> SPDControllerWithQP_Right1/10(J)
  [dt] -> SPDControllerWithQP_Right1/19(dt)
  [a_r] -> SPDControllerWithQP_Right1/20(a)
  [qdot_max_r] -> SPDControllerWithQP_Right1/13(qdot_max)
  [V_des_r] -> SPDControllerWithQP_Right1/6(Vdes)
  [TaskKv_r] -> SPDControllerWithQP_Right1/18(TaskKv)
  [TaskKp_r] -> SPDControllerWithQP_Right1/17(TaskKp)

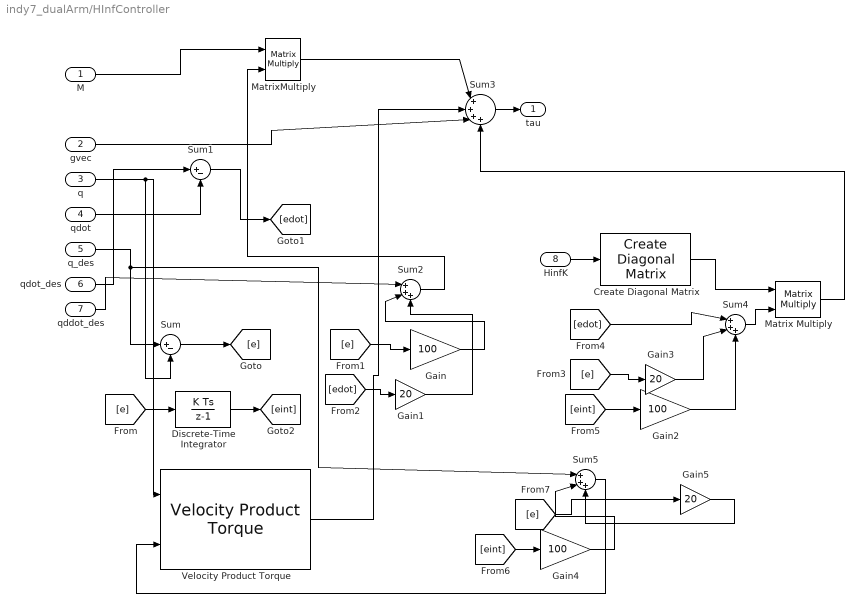
== system indy7_dualArm/HInfController ==
  M : Inport
  gvec : Inport  Port=2
  q : Inport  Port=3
  qdot : Inport  Port=4
  q_des : Inport  Port=5
  qdot_des : Inport  Port=6
  qddot_des : Inport  Port=7
  HinfK : Inport  Port=8
  Create Diagonal Matrix : matrix_library/Create Diagonal Matrix
      settings: LibrarySourceBlock=|
      | simulink/Matrix
      | Operations/Create Diagonal
      | Matrix
  Discrete-Time Integrator : DiscreteIntegrator  SampleTime=-1  LimitOutput=on  UpperSaturationLimit=10  LowerSaturationLimit=-10  ICPrevOutput=DiscIntNeverNeededParam  ICPrevScaledInput=DiscIntNeverNeededParam
  Gain : Gain  Gain=100
  Gain1 : Gain  Gain=20
  Gain2 : Gain  Gain=100
  Gain3 : Gain  Gain=20
  Gain4 : Gain  Gain=100
  Gain5 : Gain  Gain=20
  Matrix Multiply : Product  Multiplication=Matrix(*)
  MatrixMultiply : Product  Multiplication=Matrix(*)
  Sum : Sum  Inputs=|+-
  Sum1 : Sum  Inputs=|+-
  Sum2 : Sum  Inputs=|+++
  Sum3 : Sum  Inputs=|++++
  Sum4 : Sum  Inputs=|+++
  Sum5 : Sum  Inputs=|+++
  Velocity Product Torque : robotmaniplib/Velocity Product Torque  RigidBodyTree=robot  SimulateUsing=Code generation
  tau : Outport
  wires:
  q_des/1 -> Sum5/1, Sum/1
  Sum/1 -> [e]
  q/1 -> Velocity Product Torque/1, Sum/2
  qdot_des/1 -> Sum1/1
  qdot/1 -> Sum1/2
  Sum1/1 -> [edot]
  [e] -> Discrete-Time Integrator/1
  Discrete-Time Integrator/1 -> [eint]
  M/1 -> MatrixMultiply/1
  qddot_des/1 -> Sum2/1
  [e] -> Gain/1
  Gain/1 -> Sum2/2
  [edot] -> Gain1/1
  Gain1/1 -> Sum2/3
  Sum2/1 -> MatrixMultiply/2
  MatrixMultiply/1 -> Sum3/1
  gvec/1 -> Sum3/3
  [eint] -> Gain2/1
  [e] -> Gain3/1
  [edot] -> Sum4/1
  Gain3/1 -> Sum4/2
  Gain2/1 -> Sum4/3
  Sum4/1 -> Matrix Multiply/2
  HinfK/1 -> Create Diagonal Matrix/1
  Matrix Multiply/1 -> Sum3/4
  Sum3/1 -> tau/1
  [eint] -> Gain4/1
  Gain4/1 -> Sum5/2
  Gain5/1 -> Sum5/3
  [e] -> Gain5/1
  Sum5/1 -> Velocity Product Torque/2
  Velocity Product Torque/1 -> Sum3/2
  Create Diagonal Matrix/1 -> Matrix Multiply/1

== system indy7_dualArm/InverseDynamics ==
  q : Inport
  qdot : Inport  Port=2
  Gravity Torque : robotmaniplib/Gravity Torque  RigidBodyTree=robot  SimulateUsing=Code generation
  Joint Space Mass Matrix : robotmaniplib/Joint Space Mass Matrix  RigidBodyTree=robot  SimulateUsing=Code generation
  Velocity Product Torque : robotmaniplib/Velocity Product Torque  RigidBodyTree=robot  SimulateUsing=Code generation
  MassMatrix : Outport
  cvec : Outport  Port=2
  grav : Outport  Port=3
  wires:
  Velocity Product Torque/1 -> cvec/1
  Joint Space Mass Matrix/1 -> MassMatrix/1
  Gravity Torque/1 -> grav/1
  q/1 -> Velocity Product Torque/1, Gravity Torque/1, Joint Space Mass Matrix/1
  qdot/1 -> Velocity Product Torque/2

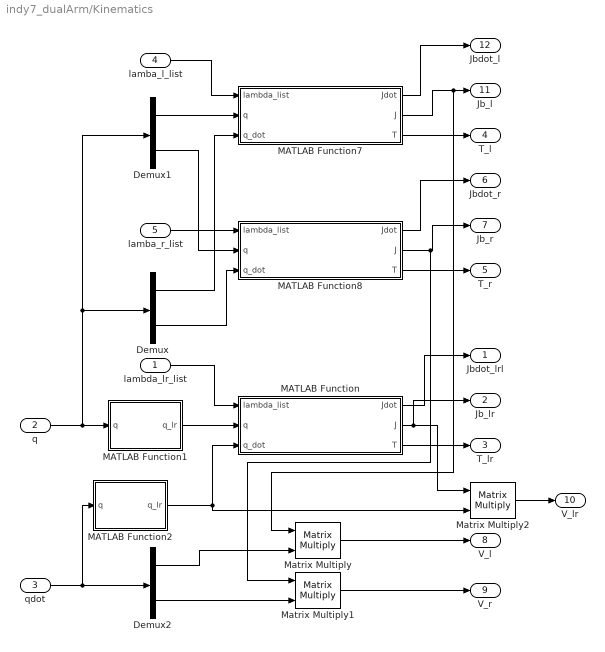
== system indy7_dualArm/Kinematics ==
  lambda_lr_list : Inport
  q : Inport  Port=2
  qdot : Inport  Port=3
  lamba_l_list : Inport  Port=4
  lamba_r_list : Inport  Port=5
  Demux : Demux  Outputs=2
  Demux1 : Demux  Outputs=2
  Demux2 : Demux  Outputs=2
  MATLAB Function : MATLAB Function  TreatAsAtomicUnit=on
  MATLAB Function1 : MATLAB Function  TreatAsAtomicUnit=on
  MATLAB Function2 : MATLAB Function  TreatAsAtomicUnit=on
  MATLAB Function7 : MATLAB Function  TreatAsAtomicUnit=on
  MATLAB Function8 : MATLAB Function  TreatAsAtomicUnit=on
  Matrix Multiply : Product  Multiplication=Matrix(*)
  Matrix Multiply1 : Product  Multiplication=Matrix(*)
  Matrix Multiply2 : Product  Multiplication=Matrix(*)
  Jbdot_lrl : Outport
  Jb_lr : Outport  Port=2
  T_lr : Outport  Port=3
  T_l : Outport  Port=4
  T_r : Outport  Port=5
  Jbdot_r : Outport  Port=6
  Jb_r : Outport  Port=7
  V_l : Outport  Port=8
  V_r : Outport  Port=9
  V_lr : Outport  Port=10
  Jb_l : Outport  Port=11
  Jbdot_l : Outport  Port=12
  wires:
  lamba_l_list/1 -> MATLAB Function7/1(lambda_list)
  MATLAB Function2/1(q_lr) -> Matrix Multiply2/2, MATLAB Function/3(q_dot)
  q/1 -> Demux1/1, Demux/1, MATLAB Function1/1(q)
  Demux/2 -> MATLAB Function8/3(q_dot)
  MATLAB Function/1(Jdot) -> Jbdot_lrl/1
  lamba_r_list/1 -> MATLAB Function8/1(lambda_list)
  Matrix Multiply/1 -> V_l/1
  Demux1/2 -> MATLAB Function8/2(q)
  qdot/1 -> Demux2/1, MATLAB Function2/1(q)
  Demux/1 -> MATLAB Function7/3(q_dot)
  Demux1/1 -> MATLAB Function7/2(q)
  lambda_lr_list/1 -> MATLAB Function/1(lambda_list)
  MATLAB Function1/1(q_lr) -> MATLAB Function/2(q)
  Demux2/1 -> Matrix Multiply/2
  Matrix Multiply1/1 -> V_r/1
  Demux2/2 -> Matrix Multiply1/2
  MATLAB Function7/1(Jdot) -> Jbdot_l/1
  MATLAB Function7/2(J) -> Matrix Multiply/1, Jb_l/1
  MATLAB Function7/3(T) -> T_l/1
  MATLAB Function8/1(Jdot) -> Jbdot_r/1
  MATLAB Function/3(T) -> T_lr/1
  MATLAB Function8/2(J) -> Matrix Multiply1/1, Jb_r/1
  MATLAB Function8/3(T) -> T_r/1
  MATLAB Function/2(J) -> Matrix Multiply2/1, Jb_lr/1
  Matrix Multiply2/1 -> V_lr/1

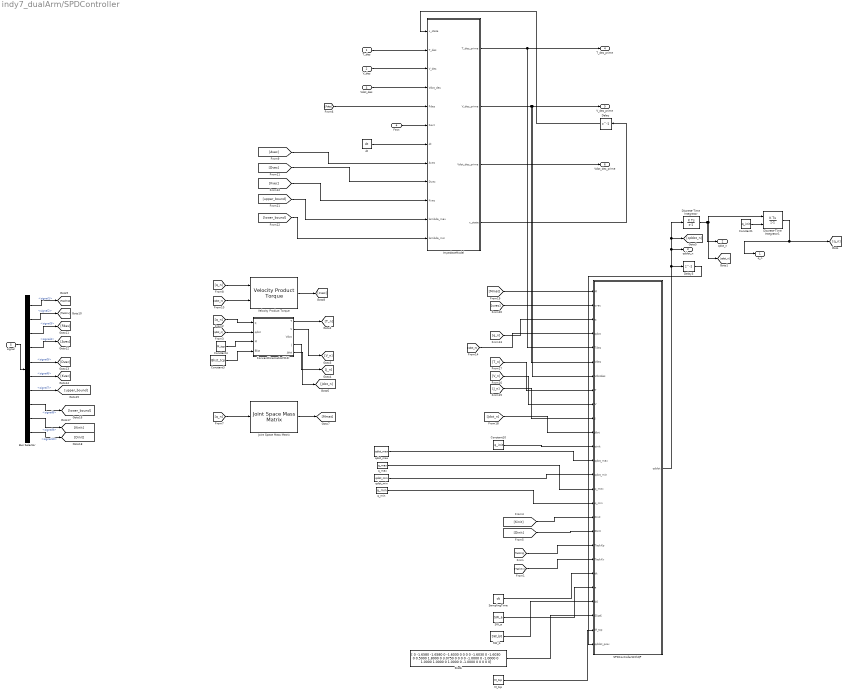
== system indy7_dualArm/SPDController ==
  T_des : Inport
  V_des : Inport  Port=2
  Vdot_des : Inport  Port=3
  Fext : Inport  Port=4
  signal : Inport  Port=5
  Bus Selector : BusSelector  OutputSignals=signal1,signal2,signal3,signal4,signal5,signal6,signal7,signal8,signal9,signal10
  Constant1 : Constant  Value=q_init  VectorParams1D=off
  Constant10 : Constant  Value=q_init  VectorParams1D=off
  Constant3 : Constant  Value=Blist_tcp
  Constant4 : Constant  Value=M_tcp
  Delay : Delay  DelayLength=1
  Delay3 : Delay  DelayLength=1
  Discrete-Time Integrator : DiscreteIntegrator  SampleTime=-1  LimitOutput=on  UpperSaturationLimit=qdot_max*1  LowerSaturationLimit=qdot_min*1  ICPrevOutput=DiscIntNeverNeededParam  ICPrevScaledInput=DiscIntNeverNeededParam
  Discrete-Time Integrator1 : DiscreteIntegrator  InitialConditionSource=external  SampleTime=-1  LimitOutput=on  UpperSaturationLimit=q_max  LowerSaturationLimit=q_min  ICPrevOutput=DiscIntNeverNeededParam  ICPrevScaledInput=DiscIntNeverNeededParam
  ForwardKinematics(510) : MATLAB Function  TreatAsAtomicUnit=on
  ImpedaceModel : MATLAB Function  TreatAsAtomicUnit=on
  Joint Space Mass Matrix : robotmaniplib/Joint Space Mass Matrix  RigidBodyTree=robot_r  SimulateUsing=Code generation
  M_tcp : Constant  Value=M_tcp
  SPDControllerWithQP : MATLAB Function  TreatAsAtomicUnit=on
  SW_a : Constant  Value=SW_a
  SW_b : Constant  Value=SW_b0
  SamplingTime : Constant  Value=dt
  Slist6 : Constant  Value=|
      | [         0   -1.6580   -1.6580         0   -1.6030         0
      |          0         0         0   -1.6030         0   -1.6030
      |          0    0.5000    1.8000         0    3.0750         0
      |          0         0         0   -1.0000         0   -1.0000
      |          0    1.0000    1.0000         0    1.0000         0
      |    -1.0000         0         0         0         0         0]
  Velocity Product Torque : robotmaniplib/Velocity Product Torque  RigidBodyTree=robot_r  SimulateUsing=Code generation
  dt : Constant  Value=dt
  q_max : Constant  Value=q_max  VectorParams1D=off
  q_min : Constant  Value=q_min  VectorParams1D=off
  qdot_max : Constant  Value=qdot_max  VectorParams1D=off
  qdot_min : Constant  Value=qdot_min  VectorParams1D=off
  q_n : Outport
  qdot_n : Outport  Port=2
  qddot_n : Outport  Port=3
  T_des_prime : Outport  Port=4
  V_des_prime : Outport  Port=5
  Vdot_des_prime : Outport  Port=6
  wires:
  M_tcp/1 -> SPDControllerWithQP/25(M_tcp)
  ImpedaceModel/4(x_state) -> Delay/1
  [Kvec] -> ImpedaceModel/10(Kvec)
  ImpedaceModel/2(V_des_prime) -> SPDControllerWithQP/7(Vdotdes), V_des_prime/1, SPDControllerWithQP/6(Vdes)
  Velocity Product Torque/1 -> [cvec]
  [q_n] -> Velocity Product Torque/1
  Constant3/1 -> ForwardKinematics(510)/4(Blist)
  [qdot_n] -> Velocity Product Torque/2
  [q_n] -> ForwardKinematics(510)/1(q)
  [qdot_n] -> ForwardKinematics(510)/2(qdot)
  Constant4/1 -> ForwardKinematics(510)/3(M)
  [q_n] -> Joint Space Mass Matrix/1
  ForwardKinematics(510)/1(T) -> [T_n]
  ForwardKinematics(510)/2(V) -> [V_n]
  ForwardKinematics(510)/4(J) -> [J_n]
  ForwardKinematics(510)/5(Jdot) -> [Jdot_n]
  Joint Space Mass Matrix/1 -> [Mmat]
  [q_n] -> SPDControllerWithQP/3(q)
  [T_n] -> SPDControllerWithQP/8(T)
  T_des/1 -> ImpedaceModel/2(T_des)
  [lower_bound] -> ImpedaceModel/12(lambda_min)
  V_des/1 -> ImpedaceModel/3(V_des)
  q_min/1 -> SPDControllerWithQP/16(q_min)
  Vdot_des/1 -> ImpedaceModel/4(Vdot_des)
  [Fdes] -> ImpedaceModel/5(Fdes)
  dt/1 -> ImpedaceModel/7(dt)
  qdot_min/1 -> SPDControllerWithQP/14(qdot_min)
  [Avec] -> ImpedaceModel/8(Avec)
  [Mmat] -> SPDControllerWithQP/1(M)
  SW_a/1 -> SPDControllerWithQP/22(a)
  [Dvec] -> ImpedaceModel/9(Dvec)
  [upper_bound] -> ImpedaceModel/11(lambda_max)
  ImpedaceModel/1(T_des_prime) -> T_des_prime/1, SPDControllerWithQP/5(Tdes)
  SamplingTime/1 -> SPDControllerWithQP/21(dt)
  ImpedaceModel/3(Vdot_des_prime) -> Vdot_des_prime/1
  Delay/1 -> ImpedaceModel/1("x_state ")
  [cvec] -> SPDControllerWithQP/2(cvec)
  [qdot_n] -> SPDControllerWithQP/4(qdot)
  [V_n] -> SPDControllerWithQP/9(V)
  [J_n] -> SPDControllerWithQP/10(J)
  [Jdot_n] -> SPDControllerWithQP/11(Jdot)
  SW_b/1 -> SPDControllerWithQP/23(b0)
  Constant10/1 -> SPDControllerWithQP/12(qinit)
  qdot_max/1 -> SPDControllerWithQP/13(qdot_max)
  q_max/1 -> SPDControllerWithQP/15(q_max)
  Slist6/1 -> SPDControllerWithQP/24(Slist6)
  SPDControllerWithQP/1(qddot) -> [qddot_n], Discrete-Time Integrator/1, qddot_n/1, Delay3/1
  Discrete-Time Integrator/1 -> [qdot_n], Discrete-Time Integrator1/1, qdot_n/1
  Delay3/1 -> SPDControllerWithQP/26(qddot_prev)
  Discrete-Time Integrator1/1 -> q_n/1, [q_n]
  Constant1/1 -> Discrete-Time Integrator1/2
  signal/1 -> Bus Selector/1
  Bus Selector/1 -> [TaskKp]  "<signal1>"
  Bus Selector/2 -> [TaskKv]  "<signal2>"
  Bus Selector/3 -> [Fdes]  "<signal3>"
  Bus Selector/4 -> [Avec]  "<signal4>"
  Bus Selector/5 -> [Dvec]  "<signal5>"
  Bus Selector/6 -> [Kvec]  "<signal6>"
  Bus Selector/7 -> [upper_bound]  "<signal7>"
  Bus Selector/8 -> [lower_bound]  "<signal8>"
  Bus Selector/9 -> [Kinit]  "<signal9>"
  Bus Selector/10 -> [Dinit]  "<signal10>"
  [TaskKp] -> SPDControllerWithQP/19(TaskKp)
  [TaskKv] -> SPDControllerWithQP/20(TaskKv)
  [Kinit] -> SPDControllerWithQP/17(Kinit)
  [Dinit] -> SPDControllerWithQP/18(Dinit)
  Fext/1 -> ImpedaceModel/6(Fext)

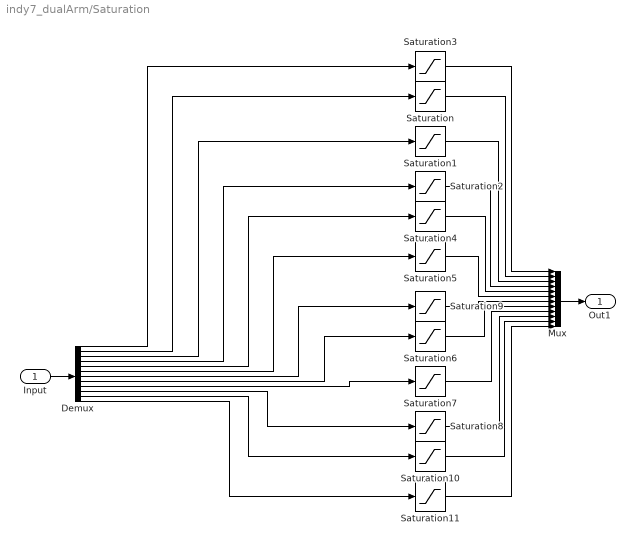
== system indy7_dualArm/Saturation ==
  Input : Inport
  Demux : Demux  Outputs=12
  Mux : Mux  Inputs=12
  Saturation{,3,6,9} (4 alike) : Saturate  UpperLimit=431.97  LowerLimit=-431.97
  Saturation1 : Saturate  UpperLimit=197.23  LowerLimit=-197.23
  Saturation{2,4..5,8,10..11} (6 alike) : Saturate  UpperLimit=79.79  LowerLimit=-79.79
  Saturation7 : Saturate  UpperLimit=197.23  LowerLimit=-197.23
  Out1 : Outport
  wires:
  Saturation9/1 -> Mux/7
  Saturation6/1 -> Mux/8
  Saturation5/1 -> Mux/6
  Saturation7/1 -> Mux/9
  Saturation4/1 -> Mux/5
  Saturation2/1 -> Mux/4
  Saturation8/1 -> Mux/10
  Saturation10/1 -> Mux/11
  Saturation1/1 -> Mux/3
  Saturation11/1 -> Mux/12
  Saturation/1 -> Mux/2
  Saturation3/1 -> Mux/1
  Demux/9 -> Saturation7/1
  Demux/10 -> Saturation8/1
  Demux/8 -> Saturation6/1
  Demux/11 -> Saturation10/1
  Demux/7 -> Saturation9/1
  Demux/12 -> Saturation11/1
  Demux/6 -> Saturation5/1
  Demux/5 -> Saturation4/1
  Demux/4 -> Saturation2/1
  Demux/3 -> Saturation1/1
  Demux/2 -> Saturation/1
  Demux/1 -> Saturation3/1
  Input/1 -> Demux/1
  Mux/1 -> Out1/1

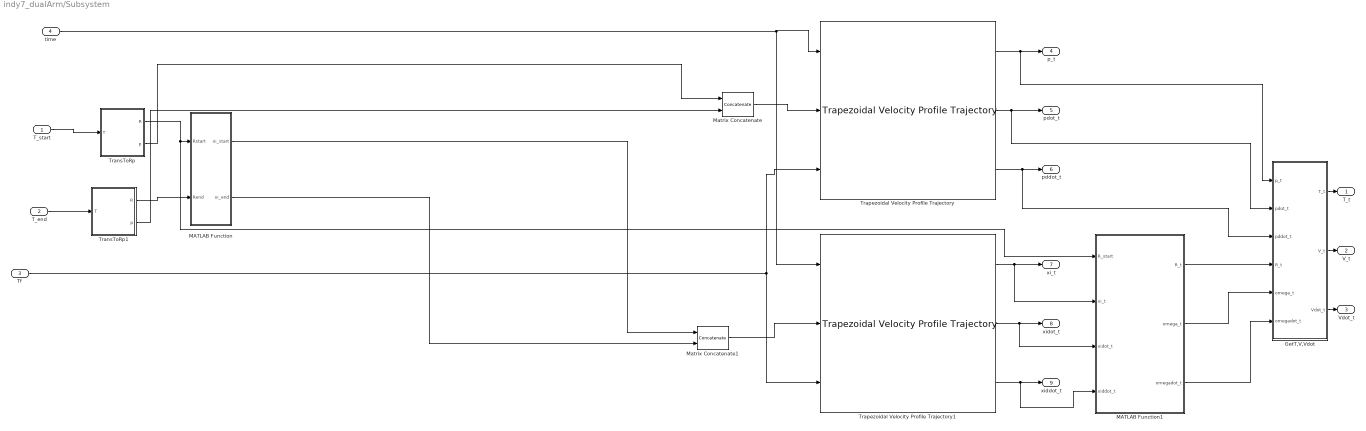
== system indy7_dualArm/Subsystem ==
  T_start : Inport
  T_end : Inport  Port=2
  Tf : Inport  Port=3
  time : Inport  Port=4
  GetT,V,Vdot : MATLAB Function  TreatAsAtomicUnit=on
  MATLAB Function : MATLAB Function  TreatAsAtomicUnit=on
  MATLAB Function1 : MATLAB Function  TreatAsAtomicUnit=on
  Matrix Concatenate : Concatenate  Mode=Multidimensional array  ConcatenateDimension=2
  Matrix Concatenate1 : Concatenate  Mode=Multidimensional array  ConcatenateDimension=2
  TransToRp : MATLAB Function  TreatAsAtomicUnit=on
  TransToRp1 : MATLAB Function  TreatAsAtomicUnit=on
  Trapezoidal Velocity Profile Trajectory : robotcorelib/Trapezoidal Velocity Profile Trajectory  WaypointSource=External  Waypoints=[ 0, -0.5, -1; 0, 0.5, 1 ]  NumParams=1  Parameter1=End Time  Parameter2=End Time  ParameterSource=External  PeakVelocity=[ 2; 2 ]  Acceleration=[ 1; 2 ]  EndTime=[ 1; 1 ]  AccelTime=[ 1; 2 ]  SimulateUsing=Code generation
  Trapezoidal Velocity Profile Trajectory1 : robotcorelib/Trapezoidal Velocity Profile Trajectory  WaypointSource=External  Waypoints=[ 0, -0.5, -1; 0, 0.5, 1 ]  NumParams=1  Parameter1=End Time  Parameter2=End Time  ParameterSource=External  PeakVelocity=[ 2; 2 ]  Acceleration=[ 1; 2 ]  EndTime=[ 1; 1 ]  AccelTime=[ 1; 2 ]  SimulateUsing=Code generation
  T_t : Outport
  V_t : Outport  Port=2
  Vdot_t : Outport  Port=3
  p_t : Outport  Port=4
  pdot_t : Outport  Port=5
  pddot_t : Outport  Port=6
  xi_t : Outport  Port=7
  xidot_t : Outport  Port=8
  xiddot_t : Outport  Port=9
  wires:
  Trapezoidal Velocity Profile Trajectory/2 -> pdot_t/1, GetT,V,Vdot/2(pdot_t)
  MATLAB Function1/2(omega_t) -> GetT,V,Vdot/5(omega_t)
  MATLAB Function1/1(R_t) -> GetT,V,Vdot/4(R_t)
  TransToRp/1(R) -> MATLAB Function1/1(R_start), MATLAB Function/1(Rstart)
  TransToRp1/2(p) -> Matrix Concatenate/2
  TransToRp/2(p) -> Matrix Concatenate/1
  Trapezoidal Velocity Profile Trajectory1/1 -> xi_t/1, MATLAB Function1/2(xi_t)
  Tf/1 -> Trapezoidal Velocity Profile Trajectory/3, Trapezoidal Velocity Profile Trajectory1/3
  MATLAB Function/1(xi_start) -> Matrix Concatenate1/1
  Trapezoidal Velocity Profile Trajectory1/3 -> xiddot_t/1, MATLAB Function1/4(xiddot_t)
  Matrix Concatenate1/1 -> Trapezoidal Velocity Profile Trajectory1/2
  Trapezoidal Velocity Profile Trajectory1/2 -> xidot_t/1, MATLAB Function1/3(xidot_t)
  MATLAB Function/2(xi_end) -> Matrix Concatenate1/2
  Matrix Concatenate/1 -> Trapezoidal Velocity Profile Trajectory/2
  T_end/1 -> TransToRp1/1(T)
  Trapezoidal Velocity Profile Trajectory/3 -> pddot_t/1, GetT,V,Vdot/3(pddot_t)
  TransToRp1/1(R) -> MATLAB Function/2(Rend)
  MATLAB Function1/3(omegadot_t) -> GetT,V,Vdot/6(omegadot_t)
  Trapezoidal Velocity Profile Trajectory/1 -> p_t/1, GetT,V,Vdot/1(p_t)
  time/1 -> Trapezoidal Velocity Profile Trajectory/1, Trapezoidal Velocity Profile Trajectory1/1
  GetT,V,Vdot/3(Vdot_t) -> Vdot_t/1
  GetT,V,Vdot/1(T_t) -> T_t/1
  GetT,V,Vdot/2(V_t) -> V_t/1
  T_start/1 -> TransToRp/1(T)

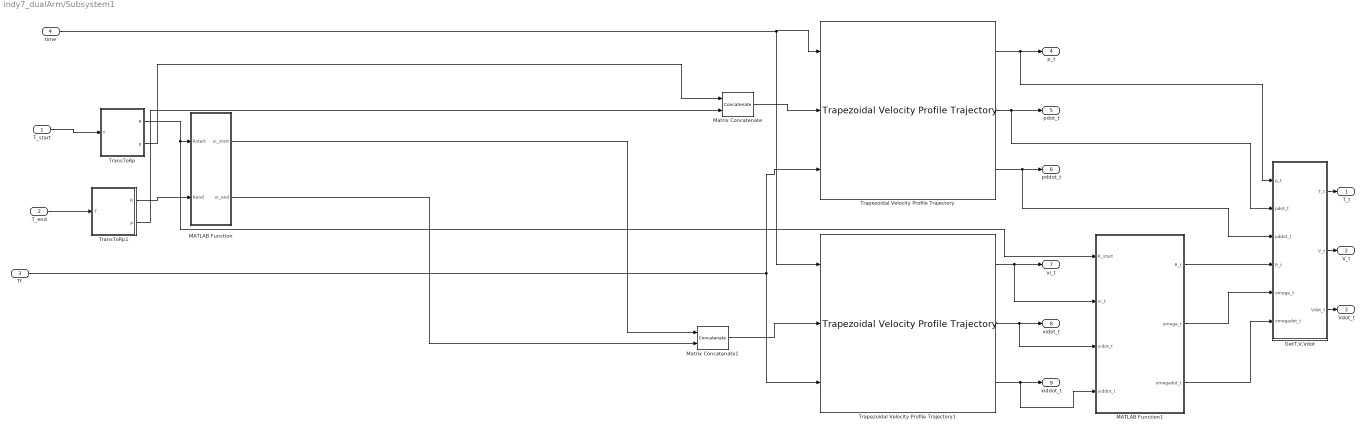
== system indy7_dualArm/Subsystem1 ==
  T_start : Inport
  T_end : Inport  Port=2
  Tf : Inport  Port=3
  time : Inport  Port=4
  GetT,V,Vdot : MATLAB Function  TreatAsAtomicUnit=on
  MATLAB Function : MATLAB Function  TreatAsAtomicUnit=on
  MATLAB Function1 : MATLAB Function  TreatAsAtomicUnit=on
  Matrix Concatenate : Concatenate  Mode=Multidimensional array  ConcatenateDimension=2
  Matrix Concatenate1 : Concatenate  Mode=Multidimensional array  ConcatenateDimension=2
  TransToRp : MATLAB Function  TreatAsAtomicUnit=on
  TransToRp1 : MATLAB Function  TreatAsAtomicUnit=on
  Trapezoidal Velocity Profile Trajectory : robotcorelib/Trapezoidal Velocity Profile Trajectory  WaypointSource=External  Waypoints=[ 0, -0.5, -1; 0, 0.5, 1 ]  NumParams=1  Parameter1=End Time  Parameter2=End Time  ParameterSource=External  PeakVelocity=[ 2; 2 ]  Acceleration=[ 1; 2 ]  EndTime=[ 1; 1 ]  AccelTime=[ 1; 2 ]  SimulateUsing=Code generation
  Trapezoidal Velocity Profile Trajectory1 : robotcorelib/Trapezoidal Velocity Profile Trajectory  WaypointSource=External  Waypoints=[ 0, -0.5, -1; 0, 0.5, 1 ]  NumParams=1  Parameter1=End Time  Parameter2=End Time  ParameterSource=External  PeakVelocity=[ 2; 2 ]  Acceleration=[ 1; 2 ]  EndTime=[ 1; 1 ]  AccelTime=[ 1; 2 ]  SimulateUsing=Code generation
  T_t : Outport
  V_t : Outport  Port=2
  Vdot_t : Outport  Port=3
  p_t : Outport  Port=4
  pdot_t : Outport  Port=5
  pddot_t : Outport  Port=6
  xi_t : Outport  Port=7
  xidot_t : Outport  Port=8
  xiddot_t : Outport  Port=9
  wires:
  Trapezoidal Velocity Profile Trajectory/2 -> pdot_t/1, GetT,V,Vdot/2(pdot_t)
  MATLAB Function1/2(omega_t) -> GetT,V,Vdot/5(omega_t)
  MATLAB Function1/1(R_t) -> GetT,V,Vdot/4(R_t)
  TransToRp/1(R) -> MATLAB Function1/1(R_start), MATLAB Function/1(Rstart)
  TransToRp1/2(p) -> Matrix Concatenate/2
  TransToRp/2(p) -> Matrix Concatenate/1
  Trapezoidal Velocity Profile Trajectory1/1 -> xi_t/1, MATLAB Function1/2(xi_t)
  Tf/1 -> Trapezoidal Velocity Profile Trajectory/3, Trapezoidal Velocity Profile Trajectory1/3
  MATLAB Function/1(xi_start) -> Matrix Concatenate1/1
  Trapezoidal Velocity Profile Trajectory1/3 -> xiddot_t/1, MATLAB Function1/4(xiddot_t)
  Matrix Concatenate1/1 -> Trapezoidal Velocity Profile Trajectory1/2
  Trapezoidal Velocity Profile Trajectory1/2 -> xidot_t/1, MATLAB Function1/3(xidot_t)
  MATLAB Function/2(xi_end) -> Matrix Concatenate1/2
  Matrix Concatenate/1 -> Trapezoidal Velocity Profile Trajectory/2
  T_end/1 -> TransToRp1/1(T)
  Trapezoidal Velocity Profile Trajectory/3 -> pddot_t/1, GetT,V,Vdot/3(pddot_t)
  TransToRp1/1(R) -> MATLAB Function/2(Rend)
  MATLAB Function1/3(omegadot_t) -> GetT,V,Vdot/6(omegadot_t)
  Trapezoidal Velocity Profile Trajectory/1 -> p_t/1, GetT,V,Vdot/1(p_t)
  time/1 -> Trapezoidal Velocity Profile Trajectory/1, Trapezoidal Velocity Profile Trajectory1/1
  GetT,V,Vdot/3(Vdot_t) -> Vdot_t/1
  GetT,V,Vdot/1(T_t) -> T_t/1
  GetT,V,Vdot/2(V_t) -> V_t/1
  T_start/1 -> TransToRp/1(T)

== system indy7_dualArm/Subsystem2 ==
  In1 : Inport
  Constant20 : Constant  Value=pi
  Demux1 : Demux  Outputs=[1,11]
  Mux1 : Mux  Inputs=[1,11]
  Sum2 : Sum  Inputs=|++
  Out1 : Outport
  wires:
  Sum2/1 -> Mux1/1
  Demux1/2 -> Mux1/2
  Constant20/1 -> Sum2/2
  In1/1 -> Demux1/1
  Demux1/1 -> Sum2/1
  Mux1/1 -> Out1/1

== system indy7_dualArm/Subsystem3 ==
  In1 : Inport
  Constant19 : Constant  Value=pi
  Demux : Demux  Outputs=[1,11]
  Mux : Mux  Inputs=[1,11]
  Sum1 : Sum  Inputs=|++
  Out1 : Outport
  wires:
  Constant19/1 -> Sum1/2
  Demux/2 -> Mux/2
  Mux/1 -> Out1/1
  In1/1 -> Demux/1
  Demux/1 -> Sum1/1
  Sum1/1 -> Mux/1
